simulink model "TeslaModelS"  (R2018b)
settings: Solver=VariableStepAuto  StartTime=0.0  StopTime=50  RelTol=1e-3
libraries: simulink x1
settings Model: Creator=Patrick  LastModifiedBy=Patrick
settings DebuggingCC: LibraryContextMissingDiagnostic=none
settings SFSimCC: SimUseLocalCustomCode=off
settings RTWCC: RTWUseLocalCustomCode=off

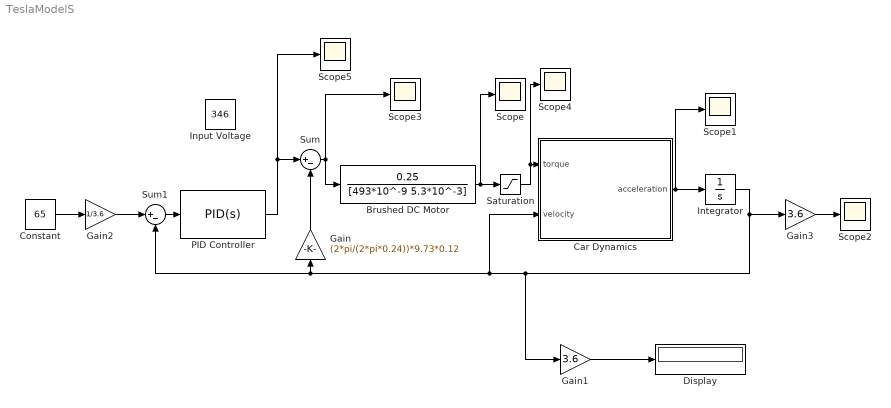
== system TeslaModelS ==
  Brushed DC Motor : TransferFcn  Numerator=[0.25]  Denominator=[493*10^-9 5.3*10^-3]
  Car Dynamics : MATLAB Function  TreatAsAtomicUnit=on
  Constant : Constant  Value=65
  Display : Display
  Gain : Gain  Gain=(2*pi/(2*pi*0.24))*9.73*0.12
  Gain1 : Gain  Gain=3.6
  Gain2 : Gain  Gain=1/3.6
  Gain3 : Gain  Gain=3.6
  Input Voltage : Constant  Value=346
  Integrator : Integrator
  PID Controller : simulink/Continuous/PID Controller  Controller=PID  Form=Parallel  TimeDomain=Continuous-time  SampleTime=-1  IntegratorMethod=Forward Euler  FilterMethod=Forward Euler  ControllerParametersSource=internal  P=50  I=3  D=100  UseFilter=on  N=100  TunerSelectOption=Transfer Function Based (PID Tuner App)  InitialConditionSource=internal  InitialConditionForIntegrator=0  InitialConditionForFilter=0  DifferentiatorICPrevScaledInput=0  ExternalReset=none  TrackingMode=off  Kt=1  LimitOutput=on  UpperSaturationLimit=346  LowerSaturationLimit=0  LinearizeAsGain=on  AntiWindupMode=none  Kb=1  POutMin=[]  POutMax=[]  IOutMin=[]  IOutMax=[]  DOutMin=[]  DOutMax=[]  NOutMin=[]  NOutMax=[]  SumOutMin=[]  SumOutMax=[]  SaturationOutMin=[]  SaturationOutMax=[]  PParamMin=[]  PParamMax=[]  IParamMin=[]  IParamMax=[]  DParamMin=[]  DParamMax=[]  NParamMin=[]  NParamMax=[]  KbParamMin=[]  KbParamMax=[]  KtParamMin=[]  KtParamMax=[]  KbOutMin=[]  KbOutMax=[]  KtOutMin=[]  KtOutMax=[]  IntegratorOutMin=[]  IntegratorOutMax=[]  FilterOutMin=[]  FilterOutMax=[]  SumI1OutMin=[]  SumI1OutMax=[]  SumI2OutMin=[]  SumI2OutMax=[]  SumI3OutMin=[]  SumI3OutMax=[]  SumI4OutMin=[]  SumI4OutMax=[]  SumDOutMin=[]  SumDOutMax=[]  DifferentiatorOutMin=[]  DifferentiatorOutMax=[]  FilterDiffOutCoefMin=[]  FilterDiffOutCoefMax=[]  ReciprocalOutMin=[]  ReciprocalOutMax=[]  SumDenOutMin=[]  SumDenOutMax=[]  SumNumOutMin=[]  SumNumOutMax=[]  DivideOutMin=[]  DivideOutMax=[]  IntegratorContinuousStateAttributes=''  IntegratorStateMustResolveToSignalObject=off  IntegratorRTWStateStorageClass=Auto  FilterContinuousStateAttributes=''  FilterStateMustResolveToSignalObject=off  FilterRTWStateStorageClass=Auto  ParallelPVariant=InternalParameters  IdealPVariant=Disabled  IVariant=InternalParameters  DVariant=InternalParameters  IntegratorVariant=Continuous  SatVariant=Enabled  AWVariant=Passthrough  PCopyVariant=Disabled  TRVariant=Disabled  FdbkBlocksVariant=Forward  IdealPFdbkVariant=Disabled  SatFdbkVariant=Disabled  DerivativeFilterVariant=ContFilter  NVariant=InternalParameters  NCopyVariant=Disabled  FilterICVariant=InternalICsFilter  IntegratorICVariant=InternalICs  ExternalResetVariant=Disabled  TRSumVariant=Passthrough  SumFdbkVariant=Disabled  SumVariant=Sum_PID
  Saturation : Saturate  UpperLimit=601  LowerLimit=0
  Scope{,1..5} (6 alike) : Scope
  Sum : Sum  Inputs=|+-
  Sum1 : Sum  Inputs=|+-
  wires:
  Gain/1 -> Sum/2
  Sum/1 -> Brushed DC Motor/1, Scope3/1
  Brushed DC Motor/1 -> Scope/1, Saturation/1
  Car Dynamics/1(acceleration) -> Scope1/1, Integrator/1
  Integrator/1 -> Gain3/1, Gain1/1, Sum1/2, Gain/1, Car Dynamics/2(velocity)
  Gain1/1 -> Display/1
  Saturation/1 -> Scope4/1, Car Dynamics/1(torque)
  PID Controller/1 -> Scope5/1, Sum/1
  Constant/1 -> Gain2/1
  Gain2/1 -> Sum1/1
  Sum1/1 -> PID Controller/1
  Gain3/1 -> Scope2/1

== matlab function TeslaModelS/Car Dynamics ==
  data: torque input; acceleration output; velocity input
function acceleration = fcn(torque, velocity)

acceleration = (40.5*torque*0.6 - 413 - 0.3381*velocity^2)/2108;
